simulink model "TI_sim_with_song"  (R2015a)
settings: Solver=ode45  StartTime=0.0  StopTime=30  RelTol=1e-3
libraries: dspvision x1, dspsnks4 x1
settings Model: Creator=ekulasek  LastModifiedBy=ekulasek

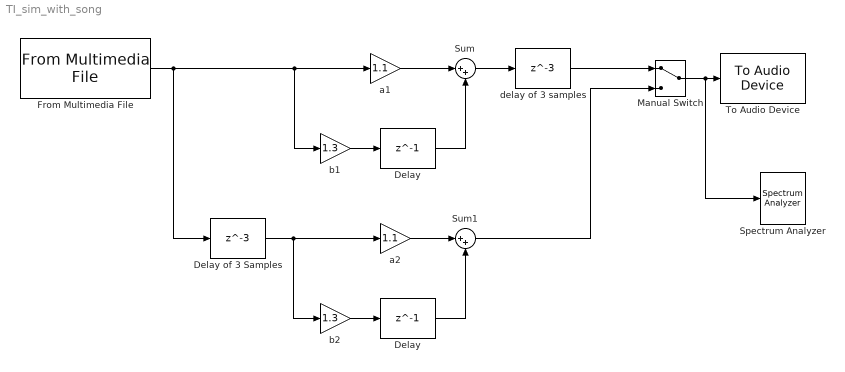
== system TI_sim_with_song ==
  Delay : Delay  DelayLength=1  InputProcessing=Columns as channels (frame based)
  "Delay " : Delay  DelayLength=1  InputProcessing=Columns as channels (frame based)
  Delay of 3 Samples : Delay  DelayLength=3  InputProcessing=Columns as channels (frame based)
  From Multimedia File : dspvision/From Multimedia File  inputFilename=/home/ekulasek/Malabe/classes/SignalsAndSystems/Programs/acappeller.wav  loop=on  numPlays=inf  outputStreams=Audio only  videoDataType=single  audioDataType=double  inheritSampleTime=on  userDefinedSampleTime=1/30  noAudioOutput=off  isIntensityVideo=off  fourcc=RGB  colorVideoFormat=Separate color signals  outputEOF=off  dataOrg=Column-major  audioFrameSize=1024  computeAudioFrameSize=off  outSamplingMode=Sample based
  Manual Switch : ManualSwitch
  Spectrum Analyzer : SpectrumAnalyzer
  Sum : Sum  Inputs=|++
  Sum1 : Sum  Inputs=|++
  To Audio Device : dspsnks4/To Audio Device  deviceName=Default  inheritSampleRate=on  sampleRate=44100  deviceDatatype=Determine from input data type  autoBufferSize=on  bufferSize=4096  queueDuration=1.0  defaultOutputChannelMapping=on  outputChannelMapping=1:2  outputNumUnderrunSamples=off
  a1 : Gain  Gain=1.1
  a2 : Gain  Gain=1.1
  b1 : Gain  Gain=1.3
  b2 : Gain  Gain=1.3
  delay of 3 samples : Delay  DelayLength=3  InputProcessing=Columns as channels (frame based)
  wires:
  a1/1 -> Sum/1
  b1/1 -> Delay/1
  Delay/1 -> Sum/2
  Sum/1 -> delay of 3 samples/1
  From Multimedia File/1 -> b1/1, a1/1, Delay of 3 Samples/1
  a2/1 -> Sum1/1
  b2/1 -> "Delay "/1
  "Delay "/1 -> Sum1/2
  Delay of 3 Samples/1 -> b2/1, a2/1
  delay of 3 samples/1 -> Manual Switch/1
  Sum1/1 -> Manual Switch/2
  Manual Switch/1 -> Spectrum Analyzer/1, To Audio Device/1
